simulink model "BLDCmotor_FOC_R2017b_fixdt"  (R2025a)
settings: Solver=FixedStepDiscrete  StartTime=0  StopTime=0.5  FixedStep=Ts  MaxStep=1e-6  RelTol=1e-6  AbsTol=1e-6  EnableMultiTasking=on
PreLoadFcn:
  | addpath(pwd);
  | addpath(genpath('01_Libraries'));
  | addpath(genpath('02_Figures'));
  | addpath(genpath('03_CreateParamTable'));
InitFcn:
  | init_model;
values from neighbouring files (symbols this model uses):
  a_cpr = 65535    [init_model.m]
  a_elecAngle = 60    [init_model.m]
  a_elecoffset = a_elecPeriod/12    (= 30)    [init_model.m]
  a_elecPeriod = 360    [init_model.m]
  a_fcpr = 1/65535    (= 1.52590218967e-05)    [init_model.m]
  a_mechoffset = a_elecoffset/n_polePairs    (= 5)    [init_model.m]
  a_phaAdvMax = 25    [init_model.m]
  b_angleMeasEna = 1    [init_model.m]
  b_cruiseCtrlEna = 0    [init_model.m]
  b_diagEna = 0    [init_model.m]
  b_fieldWeakEna = 0    [init_model.m]
  cf_currFilt = 0.692    [init_model.m]
  cf_idKi = Ki / (f_ctrl)    (= 0.00409061543436)    [init_model.m]
  cf_idKp = Kp    (= 0.0523598775598)    [init_model.m]
  cf_iqKi = Ki / (f_ctrl)    (= 0.00409061543436)    [init_model.m]
  cf_iqKiLimProt = 60 / (f_ctrl)    (= 0.00375)    [init_model.m]
  cf_iqKp = Kp    (= 0.0523598775598)    [init_model.m]
  cf_KbLimProt = Simulink.Parameter    [init_model.m]
  cf_nKi = 20.4 / (f_ctrl)    (= 0.001275)    [init_model.m]
  cf_nKiLimProt = 20 / (f_ctrl)    (= 0.00125)    [init_model.m]
  cf_nKp = 1.18    [init_model.m]
  cf_speedCoef = round(f_ctrl * a_mechAngle * (pi/180) * (30/pi))    [init_model.m]
  CTRL_FOC = 2    [init_model.m]
  CTRL_SIN = 1    [init_model.m]
  dV_openRate = 1000 / (f_ctrl)    (= 0.0625)    [init_model.m]
  dz_cntTrnsDetHi = 40    [init_model.m]
  dz_cntTrnsDetLo = 20    [init_model.m]
  ff_gain = ((r_motn / i_sca) * ((GD32_Vd_max_margin) / v_bus))    (= 0.338958333333)    [init_model.m]
  GD32_Vd_max_margin = GD32_Vd_max - V_margin    (= 1627)    [init_model.m]
  GD32_Vq_max_M1 = sqrt(GD32_Vd_max_margin^2 - GD32_Vq_max_XA.^2)    [init_model.m]
  i_max = i_max * i_sca    (= 500)    [init_model.m]
  id_fieldWeakMax = 5 * i_sca    (= 250)    [init_model.m]
  iq_maxSca_M1 = sqrt(1 - iq_maxSca_XA.^2)    [init_model.m]
  mcu_model = GD32F103    (= 1)    [init_model.m]
  n_commAcvLo = 15    [init_model.m]
  n_commDeacvHi = 30    [init_model.m]
  n_cruiseMotTgt = 0    [init_model.m]
  n_fieldWeakAuthHi = 300    [init_model.m]
  n_fieldWeakAuthLo = 100    [init_model.m]
  n_max = 1950    [init_model.m]
  n_polePairs = 6    [init_model.m]
  n_stdStillDet = 3    [init_model.m]
  OPEN_MODE = 0    [init_model.m]
  r_cos_M1 = cos((a_elecAngle_XA + a_elecPeriod/12)*(pi/180))    [init_model.m]
  r_errInpTgtThres = 600    [init_model.m]
  r_fieldWeakHi = 1000    [init_model.m]
  r_fieldWeakLo = 750    [init_model.m]
  r_motn = r_mot/2    (= 0.25)    [init_model.m]
  r_sin3PhaA_M1 = sin3Arm + A*r_sinPhaA_M1    [init_model.m]
  r_sin3PhaB_M1 = sin3Arm + A*r_sinPhaB_M1    [init_model.m]
  r_sin3PhaC_M1 = sin3Arm + A*r_sinPhaC_M1    [init_model.m]
  r_sin_M1 = sin((a_elecAngle_XA + a_elecPeriod/12)*(pi/180))    [init_model.m]
  SPD_MODE = 2    [init_model.m]
  STM32_Vd_max_margin = STM32_Vd_max - V_margin    (= 940)    [init_model.m]
  STM32_Vq_max_M1 = sqrt(STM32_Vd_max_margin^2 - STM32_Vq_max_XA.^2)    [init_model.m]
  t_errDequal = 1.80 * f_ctrl    (= 28800)    [init_model.m]
  t_errQual = 0.24 * f_ctrl    (= 3840)    [init_model.m]
  tgt_scale = 2047    [init_model.m]
  TRQ_MODE = 3    [init_model.m]
  Ts = 5e-6    (= 5e-06)    [init_model.m]
  Ts_ctrl = 6e-5    (= 6e-05)    [init_model.m]
  v_bus = 24    [init_model.m]
  vec_hallToPos = [0 2 0 1 4 3 5 0]    [init_model.m]
  VLT_MODE = 1    [init_model.m]
  z_commutMap_M1 = [-1 -1  0  1  1  0 ... (first row only)    [init_model.m]
  z_ctrlModReq = TRQ_MODE    (= 3)    [init_model.m]
  z_ctrlTypSel = CTRL_FOC    (= 2)    [init_model.m]
  z_maxCntRst = 2000    [init_model.m]
  z_selPhaCurMeasABC = 2    [init_model.m]
undefined symbols (not defined in the file or in its folder): BLDCmotor_FOC_R2017b_fixdt, DiscIntNeverNeededParam, DWORK0, DWORK1, DWORK2, DWORK3, powergui, spspowerguiLib
libraries: BLDC_controller_Lib x18, simulink x13, prociolib x6, eePwmGenerator x6, eePwmGeneratorMultilevel x3, mcbpositiondecoderlib x2, slpidlib x2, spsControlledVoltageSourceLib x1, spsMultimeterLib x1, spsPermanentMagnetSynchronousMachineLib x1, spsUniversalBridgeLib x1, spsVoltageMeasurementLib x1
(part 3 of 6)

== system BLDCmotor_FOC_R2017b_fixdt/BLDC_model_closed/__OutputSSForSFun__ ==
  __UniqueInportName__1__ : Inport
  __UniqueInportName__2__ : Inport  Port=2
  __UniqueInportName__3__ : Inport  Port=3
  __UniqueInportName__4__ : Inport  Port=4
  __UniqueInportName__5__ : Inport  Port=5
  __UniqueInportName__6__ : Inport  Port=6
  __UniqueInportName__7__ : Inport  Port=7
  __UniqueInportName__8__ : Inport  Port=8
  __UniqueInportName__9__ : Inport  Port=9
  __UniqueInportName__10__ : Inport  Port=10
  __UniqueInportName__11__ : Inport  Port=11
  __UniqueInportName__12__ : Inport  Port=12
  Mux1 : BusCreator  Inputs=12
  motor_out : Outport  VectorParamsAs1DForOutWhenUnconnected=off
  wires:
  __UniqueInportName__1__/1 -> Mux1/1  "Stator current is_a (A)"
  __UniqueInportName__2__/1 -> Mux1/2  "Stator current is_b (A)"
  __UniqueInportName__3__/1 -> Mux1/3  "Stator current is_c (A)"
  __UniqueInportName__4__/1 -> Mux1/4  "Stator back EMF e_a (V)"
  __UniqueInportName__5__/1 -> Mux1/5  "Stator back EMF e_b (V)"
  __UniqueInportName__6__/1 -> Mux1/6  "Stator back EMF e_cV)"
  __UniqueInportName__7__/1 -> Mux1/7  "Hall effect signal h_a"
  __UniqueInportName__8__/1 -> Mux1/8  "Hall effect signal h_b"
  __UniqueInportName__9__/1 -> Mux1/9  "Hall effect signal h_c"
  __UniqueInportName__10__/1 -> Mux1/10  "Rotor speed wm (rad/s)"
  __UniqueInportName__11__/1 -> Mux1/11  "Rotor angle thetam (rad)"
  __UniqueInportName__12__/1 -> Mux1/12  "Electromagnetic torque Te (N*m)"
  Mux1/1 -> motor_out/1

== system BLDCmotor_FOC_R2017b_fixdt/BLDC_model_open1/powergui ==
  note: Graphical user interface for the analysis of
      | Simscape Power Systems (Specialized Technology) circuits.
      | Place the Powergui block in the top-level of your model and double-click
      | on it to open the GUI.
  EquivalentModel1 : Subsystem
      mask init:
      | S  = GetDataForEquivalentModel('Discrete',gcbh);
      mask Display:
      | color('red')
      | disp('EQUIVALENT CIRCUIT\nDiscrete')
  Ground : Ground
  Terminator : Terminator
  wires:
  Ground/1 -> Terminator/1

== system BLDCmotor_FOC_R2017b_fixdt/PWM_gates/MCU_VD_Selector ==
  In1 : Inport
  Default_Control_Type : Subsystem
  Default_Control_Type1 : Subsystem
  If1 : If  IfExpression=u1 == 1
  Merge : Merge
  Vd_max1 : Constant  Value=GD32_Vd_max_margin  OutDataTypeStr=fixdt(1,16,4)
  Vd_max3 : Constant  Value=STM32_Vd_max_margin  OutDataTypeStr=fixdt(1,16,4)
  Out1 : Outport
  wires:
  Default_Control_Type/1(2) -> Merge/2
  Vd_max1/1 -> Default_Control_Type1/1(1)
  If1/2 -> Default_Control_Type/Action
  If1/1 -> Default_Control_Type1/Action
  Vd_max3/1 -> Default_Control_Type/1(1)
  In1/1 -> If1/1
  Merge/1 -> Out1/1
  Default_Control_Type1/1(2) -> Merge/1

== system BLDCmotor_FOC_R2017b_fixdt/PWM_gates/PWM_generator1 ==
  DC : Inport  SampleTime=Ts
  PWM_generator_sfcn : S-Function  FunctionName=PWM_generator_sf  SFunctionModules=""  SFunctionDeploymentMode=off  EnableBusSupport=off  SFcnStateName=DWORK0  mask{rtw_sf_name=PWM_generator_sf, showVar=off}
      mask prompts: rtw_sf_name "Simulink:masks:GenSFuncName_MP"; showVar "Simulink:masks:GenSFuncShowModuleList_MP"
      mask help: Simulink:masks:GenSFuncDesc_MD
      mask init: same as BLDCmotor_FOC_R2017b_fixdt/BLDC_model_closed/BLDC_model_sfcn
      settings: SFcnIsStateOwnerBlock=on
      settings: CopyFcn=|
      | if ~strcmp(get_param(gcb,'Linkstatus'),'none') && ...
      | ~strcmp(get_param(gcb,'Linkstatus'),'implicit')
      |   set_param(gcb,'LinkStatus','none');
      | end
      mask Help: eval('feval(''rtwprivate'',''rtwhelpview'',''rtw_sfcn_block'')');
      mask Display:
      | port_label('input',1,'DC');
      | port_label('output',1,'PWM');
  __InputSSForSFun__ : Subsystem
  __OutputSSForSFun__ : Subsystem
  PWM : Outport  VectorParamsAs1DForOutWhenUnconnected=off
  wires:
  __OutputSSForSFun__/1(PWM) -> PWM/1
  PWM_generator_sfcn/1 -> __OutputSSForSFun__/1(__UniqueInportName__1__)
  __InputSSForSFun__/1(__UniqueOutportName__1__) -> PWM_generator_sfcn/1
  DC/1 -> __InputSSForSFun__/1(DC)

== system BLDCmotor_FOC_R2017b_fixdt/PWM_gates/PWM_generator12 ==
  DC : Inport  SampleTime=Ts
  PWM_generator_sfcn : S-Function  FunctionName=PWM_generator_sf  SFunctionModules=""  SFunctionDeploymentMode=off  EnableBusSupport=off  SFcnStateName=DWORK0  mask{rtw_sf_name=PWM_generator_sf, showVar=off}
      mask prompts: rtw_sf_name "Simulink:masks:GenSFuncName_MP"; showVar "Simulink:masks:GenSFuncShowModuleList_MP"
      mask help: Simulink:masks:GenSFuncDesc_MD
      mask init: same as BLDCmotor_FOC_R2017b_fixdt/BLDC_model_closed/BLDC_model_sfcn
      settings: SFcnIsStateOwnerBlock=on
      settings: CopyFcn=|
      | if ~strcmp(get_param(gcb,'Linkstatus'),'none') && ...
      | ~strcmp(get_param(gcb,'Linkstatus'),'implicit')
      |   set_param(gcb,'LinkStatus','none');
      | end
      mask Help: eval('feval(''rtwprivate'',''rtwhelpview'',''rtw_sfcn_block'')');
      mask Display:
      | port_label('input',1,'DC');
      | port_label('output',1,'PWM');
  __InputSSForSFun__ : Subsystem
  __OutputSSForSFun__ : Subsystem
  PWM : Outport  VectorParamsAs1DForOutWhenUnconnected=off
  wires:
  DC/1 -> __InputSSForSFun__/1(DC)
  __InputSSForSFun__/1(__UniqueOutportName__1__) -> PWM_generator_sfcn/1
  PWM_generator_sfcn/1 -> __OutputSSForSFun__/1(__UniqueInportName__1__)
  __OutputSSForSFun__/1(PWM) -> PWM/1

== system BLDCmotor_FOC_R2017b_fixdt/PWM_gates/PWM_generator2 ==
  DC : Inport  SampleTime=Ts
  PWM_generator_sfcn : S-Function  FunctionName=PWM_generator_sf  SFunctionModules=""  SFunctionDeploymentMode=off  EnableBusSupport=off  SFcnStateName=DWORK0  mask{rtw_sf_name=PWM_generator_sf, showVar=off}
      mask prompts: rtw_sf_name "Simulink:masks:GenSFuncName_MP"; showVar "Simulink:masks:GenSFuncShowModuleList_MP"
      mask help: Simulink:masks:GenSFuncDesc_MD
      mask init: same as BLDCmotor_FOC_R2017b_fixdt/BLDC_model_closed/BLDC_model_sfcn
      settings: SFcnIsStateOwnerBlock=on
      settings: CopyFcn=|
      | if ~strcmp(get_param(gcb,'Linkstatus'),'none') && ...
      | ~strcmp(get_param(gcb,'Linkstatus'),'implicit')
      |   set_param(gcb,'LinkStatus','none');
      | end
      mask Help: eval('feval(''rtwprivate'',''rtwhelpview'',''rtw_sfcn_block'')');
      mask Display:
      | port_label('input',1,'DC');
      | port_label('output',1,'PWM');
  __InputSSForSFun__ : Subsystem
  __OutputSSForSFun__ : Subsystem
  PWM : Outport  VectorParamsAs1DForOutWhenUnconnected=off
  wires:
  DC/1 -> __InputSSForSFun__/1(DC)
  __InputSSForSFun__/1(__UniqueOutportName__1__) -> PWM_generator_sfcn/1
  PWM_generator_sfcn/1 -> __OutputSSForSFun__/1(__UniqueInportName__1__)
  __OutputSSForSFun__/1(PWM) -> PWM/1

== system BLDCmotor_FOC_R2017b_fixdt/PWM_gates/PWM_generator3 ==
  DC : Inport  SampleTime=Ts
  PWM_generator_sfcn : S-Function  FunctionName=PWM_generator_sf  SFunctionModules=""  SFunctionDeploymentMode=off  EnableBusSupport=off  SFcnStateName=DWORK0  mask{rtw_sf_name=PWM_generator_sf, showVar=off}
      mask prompts: rtw_sf_name "Simulink:masks:GenSFuncName_MP"; showVar "Simulink:masks:GenSFuncShowModuleList_MP"
      mask help: Simulink:masks:GenSFuncDesc_MD
      mask init: same as BLDCmotor_FOC_R2017b_fixdt/BLDC_model_closed/BLDC_model_sfcn
      settings: SFcnIsStateOwnerBlock=on
      settings: CopyFcn=|
      | if ~strcmp(get_param(gcb,'Linkstatus'),'none') && ...
      | ~strcmp(get_param(gcb,'Linkstatus'),'implicit')
      |   set_param(gcb,'LinkStatus','none');
      | end
      mask Help: eval('feval(''rtwprivate'',''rtwhelpview'',''rtw_sfcn_block'')');
      mask Display:
      | port_label('input',1,'DC');
      | port_label('output',1,'PWM');
  __InputSSForSFun__ : Subsystem
  __OutputSSForSFun__ : Subsystem
  PWM : Outport  VectorParamsAs1DForOutWhenUnconnected=off
  wires:
  __OutputSSForSFun__/1(PWM) -> PWM/1
  PWM_generator_sfcn/1 -> __OutputSSForSFun__/1(__UniqueInportName__1__)
  __InputSSForSFun__/1(__UniqueOutportName__1__) -> PWM_generator_sfcn/1
  DC/1 -> __InputSSForSFun__/1(DC)

== system BLDCmotor_FOC_R2017b_fixdt/PWM_gates/PWM_generator4 ==
  DC : Inport  SampleTime=Ts
  PWM_generator_sfcn : S-Function  FunctionName=PWM_generator_sf  SFunctionModules=""  SFunctionDeploymentMode=off  EnableBusSupport=off  SFcnStateName=DWORK0  mask{rtw_sf_name=PWM_generator_sf, showVar=off}
      mask prompts: rtw_sf_name "Simulink:masks:GenSFuncName_MP"; showVar "Simulink:masks:GenSFuncShowModuleList_MP"
      mask help: Simulink:masks:GenSFuncDesc_MD
      mask init: same as BLDCmotor_FOC_R2017b_fixdt/BLDC_model_closed/BLDC_model_sfcn
      settings: SFcnIsStateOwnerBlock=on
      settings: CopyFcn=|
      | if ~strcmp(get_param(gcb,'Linkstatus'),'none') && ...
      | ~strcmp(get_param(gcb,'Linkstatus'),'implicit')
      |   set_param(gcb,'LinkStatus','none');
      | end
      mask Help: eval('feval(''rtwprivate'',''rtwhelpview'',''rtw_sfcn_block'')');
      mask Display:
      | port_label('input',1,'DC');
      | port_label('output',1,'PWM');
  __InputSSForSFun__ : Subsystem
  __OutputSSForSFun__ : Subsystem
  PWM : Outport  VectorParamsAs1DForOutWhenUnconnected=off
  wires:
  DC/1 -> __InputSSForSFun__/1(DC)
  __InputSSForSFun__/1(__UniqueOutportName__1__) -> PWM_generator_sfcn/1
  PWM_generator_sfcn/1 -> __OutputSSForSFun__/1(__UniqueInportName__1__)
  __OutputSSForSFun__/1(PWM) -> PWM/1

== system BLDCmotor_FOC_R2017b_fixdt/PWM_gates/PWM_generator5 ==
  DC : Inport  SampleTime=Ts
  PWM_generator_sfcn : S-Function  FunctionName=PWM_generator_sf  SFunctionModules=""  SFunctionDeploymentMode=off  EnableBusSupport=off  SFcnStateName=DWORK0  mask{rtw_sf_name=PWM_generator_sf, showVar=off}
      mask prompts: rtw_sf_name "Simulink:masks:GenSFuncName_MP"; showVar "Simulink:masks:GenSFuncShowModuleList_MP"
      mask help: Simulink:masks:GenSFuncDesc_MD
      mask init: same as BLDCmotor_FOC_R2017b_fixdt/BLDC_model_closed/BLDC_model_sfcn
      settings: SFcnIsStateOwnerBlock=on
      settings: CopyFcn=|
      | if ~strcmp(get_param(gcb,'Linkstatus'),'none') && ...
      | ~strcmp(get_param(gcb,'Linkstatus'),'implicit')
      |   set_param(gcb,'LinkStatus','none');
      | end
      mask Help: eval('feval(''rtwprivate'',''rtwhelpview'',''rtw_sfcn_block'')');
      mask Display:
      | port_label('input',1,'DC');
      | port_label('output',1,'PWM');
  __InputSSForSFun__ : Subsystem
  __OutputSSForSFun__ : Subsystem
  PWM : Outport  VectorParamsAs1DForOutWhenUnconnected=off
  wires:
  __OutputSSForSFun__/1(PWM) -> PWM/1
  PWM_generator_sfcn/1 -> __OutputSSForSFun__/1(__UniqueInportName__1__)
  __InputSSForSFun__/1(__UniqueOutportName__1__) -> PWM_generator_sfcn/1
  DC/1 -> __InputSSForSFun__/1(DC)

== system BLDCmotor_FOC_R2017b_fixdt/PWM_gates/signal_log6 ==
  PWM : Inport
  Terminator_1 : Terminator
  wires:
  PWM/1 -> Terminator_1/1  "PWM"

== system BLDCmotor_FOC_R2017b_fixdt/Power Stage/Subsystem ==
  the : Inport
  Angle converter : spsPMSynchronousMachineModel/Discrete/Hall effect sensor/Angle converter  SystemSampleTime=-1  VariantActivationTime=update diagram  EmptyChoice=off  PassThrough=off  PassThroughVariantControl=(default)  EmptyChoiceVariantControl=(default)  AllowFlexibleInterface=on  Latency=0  AutoFrameSizeCalculation=off
  Bus Creator : BusCreator  Inputs=3
  Constant : Constant  Value=-60
  Constant1 : Constant  Value=120
  Constant2 : Constant  Value=60
  Constant3 : Constant  Value=-120
  Constant4 : Constant  Value=-180
  Constant5 : Constant  Value=0
  Data Type Conversion : DataTypeConversion  OutDataTypeStr=double
  Data Type Conversion1 : DataTypeConversion  OutDataTypeStr=double
  Data Type Conversion2 : DataTypeConversion  OutDataTypeStr=double
  Logical Operator : Logic  AllPortsSameDT=off  OutDataTypeStr=boolean
  Logical Operator1 : Logic  Operator=OR  AllPortsSameDT=off  OutDataTypeStr=boolean
  Logical Operator2 : Logic  AllPortsSameDT=off  OutDataTypeStr=boolean
  Relational Operator1 : RelationalOperator  Operator=<=
  Relational Operator2 : RelationalOperator
  Relational Operator3 : RelationalOperator  Operator=<=
  Relational Operator4 : RelationalOperator
  Relational Operator5 : RelationalOperator  Operator=<=
  Relational Operator6 : RelationalOperator
  Hall : Outport  VectorParamsAs1DForOutWhenUnconnected=off
  wires:
  Relational Operator4/1 -> Logical Operator1/1
  Constant/1 -> Relational Operator2/2
  Logical Operator/1 -> Data Type Conversion/1
  Logical Operator1/1 -> Data Type Conversion1/1
  Relational Operator5/1 -> Logical Operator2/2
  Angle converter/1 -> Relational Operator2/1, Relational Operator1/1, Relational Operator6/1, Relational Operator5/1, Relational Operator3/1, Relational Operator4/1
  Logical Operator2/1 -> Data Type Conversion2/1
  Constant2/1 -> Relational Operator4/2
  Data Type Conversion1/1 -> Bus Creator/2
  the/1 -> Angle converter/1
  Data Type Conversion/1 -> Bus Creator/1
  Constant5/1 -> Relational Operator5/2
  Data Type Conversion2/1 -> Bus Creator/3
  Relational Operator3/1 -> Logical Operator1/2
  Constant4/1 -> Relational Operator6/2
  Relational Operator1/1 -> Logical Operator/2
  Relational Operator2/1 -> Logical Operator/1
  Relational Operator6/1 -> Logical Operator2/1
  Bus Creator/1 -> Hall/1
  Constant3/1 -> Relational Operator3/2
  Constant1/1 -> Relational Operator1/2

== system BLDCmotor_FOC_R2017b_fixdt/Power Stage/Variant Subsystem ==
  note: 1) Add Subsystem or Model blocks as valid variant choices.
      | 2) You cannot connect blocks at this level. At simulation, connectivity is automatically
      | determined, based on the active variant and port name matching.
  GD32F103 : Subsystem  TreatAsAtomicUnit=on  VariantControl=mcu_model == 1
  STM32F103 : Subsystem  TreatAsAtomicUnit=on  VariantControl=mcu_model == 0
  Vd_max_margin : Outport

== system BLDCmotor_FOC_R2017b_fixdt/filtLowPass/Low_Pass_Filter ==
  u : Inport
  coef : Inport  Port=2
  Divide3 : Product  Inputs=**  OutDataTypeStr=fixdt(1,32,16)  RndMeth=Simplest  SaturateOnIntegerOverflow=on
  Scope1 : Scope  NumInputPorts=3
      settings: ActiveDisplayYMinimum=-7973.4546189633093  ActiveDisplayYMaximum=13277.671743224013
  Sum2 : Sum  Inputs=+-  RndMeth=Simplest
  Sum3 : Sum  RndMeth=Simplest  OutDataTypeStr=Inherit: Same as first input
  UnitDelay1 : UnitDelay  SampleTime=-1  HasFrameUpgradeWarning=on
  y : Outport  VectorParamsAs1DForOutWhenUnconnected=off
  wires:
  Divide3/1 -> Scope1/2, Sum3/1
  Sum3/1 -> y/1, Scope1/3, UnitDelay1/1
  UnitDelay1/1 -> Sum3/2, Sum2/2
  Sum2/1 -> Divide3/1, Scope1/1
  u/1 -> Sum2/1
  coef/1 -> Divide3/2

== system BLDCmotor_FOC_R2017b_fixdt/rateLimiter/Rate_Limiter ==
  note: Rate Limiter
      | Note: The sample time must be included in the Increment and Decrement values.
  u : Inport
  inc : Inport  Port=2
  dec : Inport  Port=3
  Saturation Dynamic : simulink/Discontinuities/Saturation Dynamic  OutMin=[]  OutMax=[]  OutDataTypeStr=Inherit: Same as second input  OutDataType=fixdt(1, 16)  OutScaling=2^-10  DoSatur=off
  Sum1 : Sum  Inputs=+-  RndMeth=Zero  OutDataTypeStr=Inherit: Same as first input
  Sum2 : Sum  RndMeth=Zero  OutDataTypeStr=Inherit: Same as first input
  UnitDelay : UnitDelay  SampleTime=-1  HasFrameUpgradeWarning=on
      settings: AttributesFormatString=Ini=%<X0>
  y : Outport  VectorParamsAs1DForOutWhenUnconnected=off
  wires:
  Saturation Dynamic/1 -> Sum2/1
  dec/1 -> Saturation Dynamic/3
  Sum1/1 -> Saturation Dynamic/2
  Sum2/1 -> UnitDelay/1, y/1
  inc/1 -> Saturation Dynamic/1
  u/1 -> Sum1/1
  UnitDelay/1 -> Sum2/2, Sum1/2

== system BLDCmotor_FOC_R2017b_fixdt/BLDC_controller/F01_Estimations/F01_01_Edge_Detector ==
  b_hallA : Inport
  b_hallB : Inport  Port=2
  b_hallC : Inport  Port=3
  Logical Operator : Logic  Operator=XOR  Inputs=6  AllPortsSameDT=off  OutDataTypeStr=boolean
  UnitDelay1 : UnitDelay  SampleTime=-1  HasFrameUpgradeWarning=on
      settings: AttributesFormatString=Ini=%<X0>
  UnitDelay2 : UnitDelay  SampleTime=-1  HasFrameUpgradeWarning=on
      settings: AttributesFormatString=Ini=%<X0>
  UnitDelay3 : UnitDelay  SampleTime=-1  HasFrameUpgradeWarning=on
      settings: AttributesFormatString=Ini=%<X0>
  "b_edge " : Outport  OutputWhenDisabled=reset  InitialOutput=0  VectorParamsAs1DForOutWhenUnconnected=off
  wires:
  b_hallA/1 -> Logical Operator/1, UnitDelay3/1
  b_hallC/1 -> Logical Operator/3, UnitDelay2/1
  b_hallB/1 -> Logical Operator/2, UnitDelay1/1
  UnitDelay1/1 -> Logical Operator/5
  UnitDelay2/1 -> Logical Operator/6
  UnitDelay3/1 -> Logical Operator/4
  Logical Operator/1 -> "b_edge "/1

== system BLDCmotor_FOC_R2017b_fixdt/BLDC_controller/F01_Estimations/F01_02_Position_Calculation ==
  note: This calculates the low resolution position based on Hall sensors.
  b_hallA : Inport
  b_hallB : Inport  Port=2
  b_hallC : Inport  Port=3
  Selector : Selector  IndexMode=Zero-based  InputPortWidth=length(vec_hallToPos)  IndexOptions=Index vector (port)  Indices=[1 3]  OutputSizes=1
  Sum : Sum  Inputs=+++  RndMeth=Simplest  OutDataTypeStr=Inherit: Same as first input
  g_Ha : Gain  Gain=4  OutDataTypeStr=Inherit: Inherit via back propagation  RndMeth=Zero  ParamDataTypeStr=Inherit: Same as input
  g_Hb : Gain  Gain=2  OutDataTypeStr=Inherit: Inherit via back propagation  RndMeth=Simplest  ParamDataTypeStr=Inherit: Same as input
  vec_hallToPos : Constant  Value=vec_hallToPos  OutDataTypeStr=int8
  z_posRaw : Outport  OutputWhenDisabled=reset  InitialOutput=0  VectorParamsAs1DForOutWhenUnconnected=off
  "z_pos " : Outport  Port=2  OutputWhenDisabled=reset  InitialOutput=0  VectorParamsAs1DForOutWhenUnconnected=off
  wires:
  b_hallC/1 -> Sum/3
  g_Ha/1 -> Sum/1
  g_Hb/1 -> Sum/2
  Sum/1 -> z_posRaw/1, Selector/2
  b_hallA/1 -> g_Ha/1
  b_hallB/1 -> g_Hb/1
  vec_hallToPos/1 -> Selector/1
  Selector/1 -> "z_pos "/1

== system BLDCmotor_FOC_R2017b_fixdt/BLDC_controller/F01_Estimations/F01_03_Direction_Detection ==
  z_pos : Inport
  Action Port : ActionPort  ActionPortLabel=if(u1 ~= 0)
  Constant20 : Constant  Value=-5  OutDataTypeStr=Inherit: Inherit via back propagation
  Constant23 : Constant  Value=-1  OutDataTypeStr=int8
  Constant24 : Constant  OutDataTypeStr=int8
  Constant8 : Constant  OutDataTypeStr=Inherit: Inherit via back propagation
  Logical Operator3 : Logic  Operator=OR  AllPortsSameDT=off  OutDataTypeStr=boolean
  Relational Operator1 : RelationalOperator  Operator===  OutDataTypeStr=boolean  RndMeth=Simplest  InputSameDT=off
  Relational Operator6 : RelationalOperator  Operator===  OutDataTypeStr=boolean  RndMeth=Simplest  InputSameDT=off
  Sum2 : Sum  Inputs=|+-  InputSameDT=on  RndMeth=Zero  OutDataTypeStr=Inherit: Same as first input
  Switch2 : Switch  Criteria=u2 ~= 0  OutDataTypeStr=Inherit: Inherit via back propagation  RndMeth=Simplest  SaturateOnIntegerOverflow=off  InputSameDT=off
  UnitDelay2 : UnitDelay  SampleTime=-1  HasFrameUpgradeWarning=on
  UnitDelay3 : UnitDelay  SampleTime=-1  HasFrameUpgradeWarning=on
      settings: AttributesFormatString=Ini=%<X0>
  z_dir : Outport  VectorParamsAs1DForOutWhenUnconnected=off
  z_dirPrev : Outport  Port=2  VectorParamsAs1DForOutWhenUnconnected=off
  wires:
  UnitDelay2/1 -> Sum2/2
  Relational Operator1/1 -> Logical Operator3/1
  Constant8/1 -> Relational Operator1/2
  Sum2/1 -> Relational Operator6/1, Relational Operator1/1
  Relational Operator6/1 -> Logical Operator3/2
  Constant20/1 -> Relational Operator6/2
  Constant24/1 -> Switch2/1
  Constant23/1 -> Switch2/3
  Logical Operator3/1 -> Switch2/2
  z_pos/1 -> Sum2/1, UnitDelay2/1
  Switch2/1 -> UnitDelay3/1, z_dir/1
  UnitDelay3/1 -> z_dirPrev/1

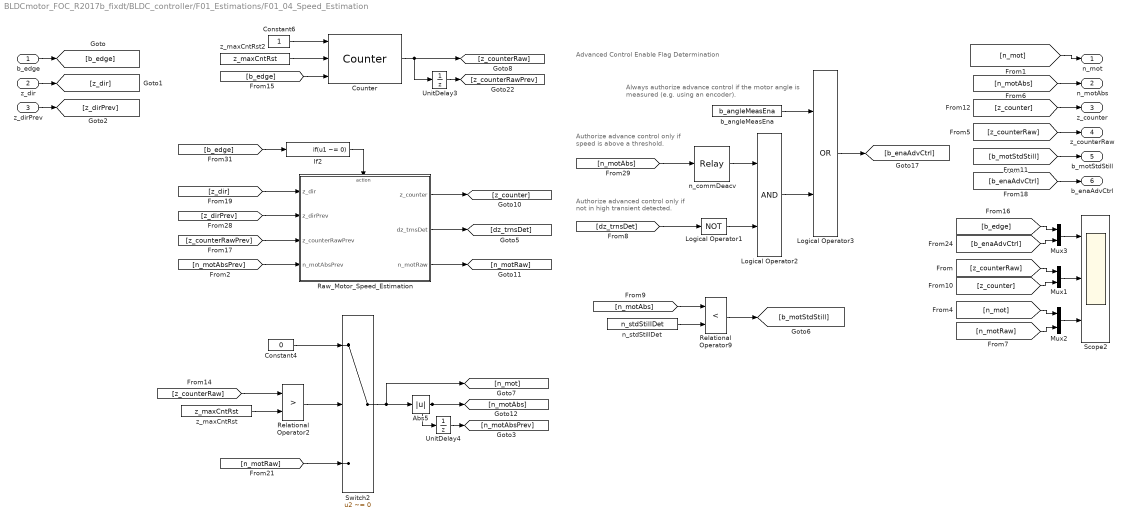
== system BLDCmotor_FOC_R2017b_fixdt/BLDC_controller/F01_Estimations/F01_04_Speed_Estimation ==
  note: Advanced Control Enable Flag Determination
  note: Authorize advance control only if speed is above a threshold.
  note: Authorize advanced control only if not in high transient detected.
  note: Always authorize advance control if the motor angle is measured (e.g. using an encoder).
  b_edge : Inport
  z_dir : Inport  Port=2
  z_dirPrev : Inport  Port=3
  Abs5 : Abs  OutDataTypeStr=Inherit: Inherit via back propagation  RndMeth=Zero  SaturateOnIntegerOverflow=off
  Constant4 : Constant  Value=0  OutDataTypeStr=Inherit: Inherit via back propagation
  Constant6 : Constant  OutDataTypeStr=fixdt(1,16,0)
  Counter : BLDC_controller_Lib/Counter  z_cntInit=z_maxCntRst
      settings: AttributesFormatString=Ini=%<z_cntInit>
  If2 : If  IfExpression=u1 ~= 0  ShowElse=off
  Logical Operator1 : Logic  Operator=NOT  AllPortsSameDT=off  OutDataTypeStr=boolean
  Logical Operator2 : Logic  AllPortsSameDT=off  OutDataTypeStr=boolean
  Logical Operator3 : Logic  Operator=OR  AllPortsSameDT=off  OutDataTypeStr=boolean
  Mux1 : Mux  Inputs=2
  Mux2 : Mux  Inputs=2
  Mux3 : Mux  Inputs=2
  Raw_Motor_Speed_Estimation : Subsystem
  Relational Operator2 : RelationalOperator  Operator=>  OutDataTypeStr=boolean  RndMeth=Simplest  InputSameDT=off
  Relational Operator9 : RelationalOperator  Operator=<  OutDataTypeStr=boolean  RndMeth=Simplest  InputSameDT=off
  Scope2 : Scope  NumInputPorts=3
      settings: ActiveDisplayYMinimum=-0.12499999999999997  ActiveDisplayYMaximum=1.125
  Switch2 : Switch  Criteria=u2 ~= 0  OutDataTypeStr=Inherit: Inherit via back propagation  RndMeth=Zero  SaturateOnIntegerOverflow=off  InputSameDT=off
  UnitDelay3 : UnitDelay  InitialCondition=z_maxCntRst  SampleTime=-1  HasFrameUpgradeWarning=on
      settings: AttributesFormatString=Ini=%<X0>
  UnitDelay4 : UnitDelay  SampleTime=-1  HasFrameUpgradeWarning=on
      settings: AttributesFormatString=Ini=%<X0>
  b_angleMeasEna : Constant  Value=b_angleMeasEna  OutDataTypeStr=boolean
  n_commDeacv : Relay  OnSwitchValue=n_commDeacvHi  OffSwitchValue=n_commAcvLo  OutDataTypeStr=boolean
  n_stdStillDet : Constant  Value=n_stdStillDet  OutDataTypeStr=Inherit: Inherit via back propagation
  z_maxCntRst : Constant  Value=z_maxCntRst  OutDataTypeStr=Inherit: Inherit via back propagation
  z_maxCntRst2 : Constant  Value=z_maxCntRst  OutDataTypeStr=Inherit: Inherit via back propagation
  n_mot : Outport  VectorParamsAs1DForOutWhenUnconnected=off
  n_motAbs : Outport  Port=2  VectorParamsAs1DForOutWhenUnconnected=off
  z_counter : Outport  Port=3  OutputWhenDisabled=reset  InitialOutput=0  VectorParamsAs1DForOutWhenUnconnected=off
  z_counterRaw : Outport  Port=4  OutputWhenDisabled=reset  InitialOutput=0  VectorParamsAs1DForOutWhenUnconnected=off
  b_motStdStill : Outport  Port=5  OutputWhenDisabled=reset  InitialOutput=0  VectorParamsAs1DForOutWhenUnconnected=off
  b_enaAdvCtrl : Outport  Port=6  VectorParamsAs1DForOutWhenUnconnected=off
  wires:
  [n_motRaw] -> Mux2/2
  Mux2/1 -> Scope2/3
  [n_mot] -> Mux2/1
  Mux1/1 -> Scope2/2
  [z_counterRaw] -> Mux1/1
  [z_counter] -> Mux1/2
  b_edge/1 -> [b_edge]
  [n_mot] -> n_mot/1
  z_dir/1 -> [z_dir]
  [z_counter] -> z_counter/1
  [z_counterRaw] -> z_counterRaw/1
  UnitDelay3/1 -> [z_counterRawPrev]
  z_dirPrev/1 -> [z_dirPrev]
  [z_dir] -> Raw_Motor_Speed_Estimation/1(z_dir)
  Abs5/1 -> UnitDelay4/1, [n_motAbs]
  Raw_Motor_Speed_Estimation/1(z_counter) -> [z_counter]
  [z_dirPrev] -> Raw_Motor_Speed_Estimation/2(z_dirPrev)
  If2/1 -> Raw_Motor_Speed_Estimation/Action
  [z_counterRawPrev] -> Raw_Motor_Speed_Estimation/3(z_counterRawPrev)
  [b_enaAdvCtrl] -> b_enaAdvCtrl/1
  [z_counterRaw] -> Relational Operator2/1
  z_maxCntRst/1 -> Relational Operator2/2
  Constant4/1 -> Switch2/1
  Raw_Motor_Speed_Estimation/3(n_motRaw) -> [n_motRaw]
  Switch2/1 -> [n_mot], Abs5/1
  Mux3/1 -> Scope2/1
  [b_enaAdvCtrl] -> Mux3/2
  [b_edge] -> Mux3/1
  [b_edge] -> If2/1
  Relational Operator2/1 -> Switch2/2
  UnitDelay4/1 -> [n_motAbsPrev]
  [n_motAbsPrev] -> Raw_Motor_Speed_Estimation/4(n_motAbsPrev)
  [n_motAbs] -> n_motAbs/1
  [n_motAbs] -> n_commDeacv/1
  Raw_Motor_Speed_Estimation/2(dz_trnsDet) -> [dz_trnsDet]
  n_commDeacv/1 -> Logical Operator2/1
  Logical Operator1/1 -> Logical Operator2/2
  [dz_trnsDet] -> Logical Operator1/1
  z_maxCntRst2/1 -> Counter/2
  [b_edge] -> Counter/3
  Constant6/1 -> Counter/1
  Counter/1 -> UnitDelay3/1, [z_counterRaw]
  [b_motStdStill] -> b_motStdStill/1
  [n_motAbs] -> Relational Operator9/1
  n_stdStillDet/1 -> Relational Operator9/2
  Relational Operator9/1 -> [b_motStdStill]
  [n_motRaw] -> Switch2/3
  Logical Operator3/1 -> [b_enaAdvCtrl]
  Logical Operator2/1 -> Logical Operator3/2
  b_angleMeasEna/1 -> Logical Operator3/1

== system BLDCmotor_FOC_R2017b_fixdt/BLDC_controller/F01_Estimations/F01_05_Electrical_Angle_Estimation ==
  note: Electrical angle calculation
  note: This switch is to manage the situation when FOC control method is not enabled.
  note: Electrical angle calculation:
      | a_elecAngle = a_elecAngle_C * (z_posLowRes + z_dir * (z_counterRaw / z_counter))
      | where a_elecAngle_C = 60
      | The min, max are for protection against angle overflow.
  z_pos : Inport
  z_dir : Inport  Port=2
  z_counter : Inport  Port=3
  z_counterRaw : Inport  Port=4
  b_enaAdvCtrl : Inport  Port=5
  Action Port : ActionPort  ActionPortLabel=if(u1 == 0)
  Constant1 : Constant  Value=0  OutDataTypeStr=Inherit: Inherit via back propagation
  Constant16 : Constant  OutDataTypeStr=Inherit: Inherit via back propagation
  Constant2 : Constant  OutDataTypeStr=Inherit: Inherit via back propagation
  Divide1 : Product  Inputs=*/  OutDataTypeStr=fixdt(1,16,14)  RndMeth=Simplest
  Divide2 : Product  Inputs=**  RndMeth=Simplest  OutDataTypeStr=Inherit: Same as first input
  Divide3 : Product  Inputs=**  RndMeth=Simplest  OutDataTypeStr=Inherit: Same as first input
  MinMax : MinMax  Inputs=2
  MinMax1 : MinMax  Function=max  Inputs=2
  Relational Operator7 : RelationalOperator  Operator===  OutDataTypeStr=boolean  RndMeth=Simplest  InputSameDT=off
  Scope : Scope  NumInputPorts=3
      settings: ActiveDisplayYMinimum=-45  ActiveDisplayYMaximum=405
  Signal Conversion2 : SignalConversion  OverrideOpt=off
  Sum1 : Sum  RndMeth=Simplest  OutDataTypeStr=Inherit: Same as first input
  Sum3 : Sum  OutDataTypeStr=fixdt(1,16,12)  RndMeth=Simplest
  Switch2 : Switch  Criteria=u2 ~= 0  OutDataTypeStr=Inherit: Inherit via back propagation  RndMeth=Zero  SaturateOnIntegerOverflow=off  InputSameDT=off
  Switch3 : Switch  Criteria=u2 ~= 0  OutDataTypeStr=Inherit: Inherit via back propagation  RndMeth=Zero  SaturateOnIntegerOverflow=off  InputSameDT=off
  a_elecAngle1 : Constant  Value=a_elecAngle  OutDataTypeStr=Inherit: Inherit via back propagation
  a_elecAngle : Outport  VectorParamsAs1DForOutWhenUnconnected=off
  wires:
  z_pos/1 -> [z_pos]
  z_dir/1 -> [z_dir]
  [a_elecAngle] -> Scope/1
  [b_enaAdvCtrl] -> Scope/3
  z_counterRaw/1 -> [z_counterRaw]
  z_counter/1 -> [z_counter]
  [z_pos] -> Switch3/1, Sum1/1
  Constant2/1 -> Sum1/2
  Relational Operator7/1 -> Switch3/2
  Constant16/1 -> Relational Operator7/2
  [z_dir] -> Relational Operator7/1
  Sum1/1 -> Switch3/3
  b_enaAdvCtrl/1 -> [b_enaAdvCtrl]
  [a_elecAngle] -> Signal Conversion2/1
  a_elecAngle1/1 -> Divide2/1
  [b_enaAdvCtrl] -> Switch2/2
  Sum3/1 -> [z_posHighRes], Switch2/1
  Divide3/1 -> Sum3/1
  Divide2/1 -> [a_elecAngle]
  [z_posLowRes] -> Sum3/2, Switch2/3
  Switch3/1 -> [z_posLowRes]
  [z_posHighRes] -> Scope/2
  Divide1/1 -> Divide3/1
  [z_dir] -> Divide3/2
  MinMax/1 -> Divide1/1
  [z_counterRaw] -> MinMax/1
  [z_counter] -> MinMax/2, Divide1/2
  Switch2/1 -> MinMax1/1
  Constant1/1 -> MinMax1/2
  MinMax1/1 -> Divide2/2
  Signal Conversion2/1 -> a_elecAngle/1

== system BLDCmotor_FOC_R2017b_fixdt/BLDC_controller/F01_Estimations/F01_06_Electrical_Angle_Measurement ==
  note: Shift angle with -30 deg to match the sin, cos look-up tables.
  note: Electrical angle calculation
  a_encoderCNT : Inport
  a_mechangle : Inport  Port=2
  Action Port : ActionPort  ActionPortLabel=else
  Constant : Constant  Value=a_cpr  OutDataTypeStr=fixdt(0,16,0)
  Constant1 : Constant  Value=a_mechoffset  OutDataTypeStr=uint16
  Constant2 : Constant  Commented=on  Value=a_elecoffset  OutDataTypeStr=Inherit: Inherit via back propagation
  Constant3 : Constant  Value=a_fcpr  OutDataTypeStr=fixdt(0,32,32)
  Data Type Conversion1 : DataTypeConversion  Commented=on  OutDataTypeStr=fixdt(0,16,0)  SaturateOnIntegerOverflow=off  RndMeth=Floor
  Data Type Conversion20 : DataTypeConversion  Commented=on  OutDataTypeStr=fixdt(1,16,6)  SaturateOnIntegerOverflow=off  RndMeth=Floor
  Divide : Product  Commented=on  Inputs=**
  From1 : From  Commented=on  GotoTag=a_mechangle
  Goto2 : Goto  Commented=on  GotoTag=a_mechangle
  Goto3 : Goto  Commented=on  GotoTag=a_elecAngle
  MechElec : Scope  NumInputPorts=7
      settings: ActiveDisplayYMinimum=-225.99465496649157  ActiveDisplayYMaximum=1430.7297186223789  DataLoggingVariableName=ScopeData4
  Mechanical to Electrical Position : mcbpositiondecoderlib/Mechanical to Electrical Position  PolePairsInputType=Input port  NrPP=n_polePairs  selectedRange=Degrees  MechOfstInputType=Input port  mechOffsetIn=a_mechoffset  maxAngleIn=360  InputDataType=fixdt(0,16,7)  VariantSelect=floating-point
      settings: LibrarySourceBlock=mcblib/Sensor Decoders/Mechanical to Electrical Position
  Modulo_fixdt : BLDC_controller_Lib/Modulo_fixdt  Commented=on  SystemSampleTime=-1  VariantActivationTime=update diagram  EmptyChoice=off  PassThrough=off  PassThroughVariantControl=(default)  EmptyChoiceVariantControl=(default)  AllowFlexibleInterface=on  Latency=0  AutoFrameSizeCalculation=off
  Quadrature Decoder : mcbpositiondecoderlib/Quadrature Decoder  ParameterInputType=on  CountsPerRevInverseDataType=fixdt(0,32,32)  EncoderSlitsPerRevolution=a_cpr  EncoderCountsPerSlit=1  CounterSize=16 bits  ExternalIndexCount=off  PositionUnit=Degrees  PositionDataType=fixdt(0,16,7)
      settings: LibrarySourceBlock=mcblib/Sensor Decoders/Quadrature Decoder
  Sum1 : Sum  Commented=on  Inputs=+-  RndMeth=Simplest  OutDataTypeStr=Inherit: Same as first input
  a_elecPeriod : Constant  Commented=on  Value=a_elecPeriod  OutDataTypeStr=Inherit: Inherit via back propagation
  n_polePairs : Constant  Commented=on  Value=n_polePairs  OutDataTypeStr=uint8
  n_polePairs1 : Constant  Value=n_polePairs  OutDataTypeStr=uint16
  a_elecAngle : Outport  VectorParamsAs1DForOutWhenUnconnected=off
  wires:
  [a_elecAngle] -> a_elecAngle/1
  a_encoderCNT/1 -> [a_encoderCNT]
  n_polePairs/1 -> Divide/2
  a_elecPeriod/1 -> Modulo_fixdt/2
  Constant2/1 -> Sum1/2
  Divide/1 -> Sum1/1
  Sum1/1 -> MechElec/4, Modulo_fixdt/1
  Modulo_fixdt/1 -> MechElec/3, Data Type Conversion20/1
  Quadrature Decoder/1 -> Mechanical to Electrical Position/1, MechElec/5
  From1/1 -> Divide/1, MechElec/1
  [a_encoderCNT] -> MechElec/7, Quadrature Decoder/1
  n_polePairs1/1 -> Mechanical to Electrical Position/2
  Mechanical to Electrical Position/1 -> MechElec/6, [a_elecAngle]
  a_mechangle/1 -> Goto2/1
  Data Type Conversion20/1 -> Goto3/1, MechElec/2
  Constant1/1 -> Mechanical to Electrical Position/3
  Constant/1 -> Quadrature Decoder/2
  Constant3/1 -> Quadrature Decoder/3

== system BLDCmotor_FOC_R2017b_fixdt/BLDC_controller/F02_Diagnostics/Diagnostics_Enabled ==
  note: Error 001: Hall sensor not connected
  note: Error 002: Hall sensor short circuit
  note: Error Qualification
  note: Error Detection
  note: Error Reporting
  note: Error 004: Motor NOT able to spin.
      |
      | Possible causes:
      | - motor phase disconnected
      | - MOSFET defective
      | - Operational Amplifier defective
      | - motor blocked
  note: This switch makes sure that once this error is SET, it can only be erased by a board restart cycle.
  note: If the Voltage applied to the motor is above a threshold but the motor does NOT spin, then there is an error.
      | Note: The error is checked only if the motor is Enabled. If it is Disabled it will not spin anyway.
  b_motEna : Inport
  z_posRaw : Inport  Port=2
  b_motStdStill : Inport  Port=3
  VqFinPrev : Inport  Port=4
  Action Port : ActionPort  ActionPortLabel=if(u1 ~= 0)
  Abs4 : Abs  SaturateOnIntegerOverflow=off
  Bitwise Operator1 : simulink/Logic and Bit Operations/Bitwise Operator  logicop=AND  UseBitMask=on  BitMask=bin2dec('100')  BitMaskRealWorld=Stored Integer
  CTRL_COMM : Constant  Value=0  OutDataTypeStr=Inherit: Inherit via back propagation
  CTRL_COMM1 : Constant  Value=7  OutDataTypeStr=Inherit: Inherit via back propagation
  CTRL_COMM2 : Constant  Value=0  OutDataTypeStr=Inherit: Inherit via back propagation
  CTRL_COMM4 : Constant  OutDataTypeStr=Inherit: Inherit via back propagation
  Data Type Conversion : DataTypeConversion  OutDataTypeStr=uint8  SaturateOnIntegerOverflow=off  RndMeth=Floor
  Data Type Conversion1 : DataTypeConversion  OutDataTypeStr=uint8  SaturateOnIntegerOverflow=off  RndMeth=Floor
  Data Type Conversion3 : DataTypeConversion  OutDataTypeStr=uint8  SaturateOnIntegerOverflow=off  RndMeth=Floor
  Debounce_Filter : BLDC_controller_Lib/Debounce_Filter
  Logical Operator1 : Logic  Inputs=3  AllPortsSameDT=off  OutDataTypeStr=boolean
  Relational Operator1 : RelationalOperator  Operator===  OutDataTypeStr=boolean  RndMeth=Simplest  InputSameDT=off
  Relational Operator2 : RelationalOperator  Operator=~=  OutDataTypeStr=boolean  RndMeth=Simplest  InputSameDT=off
  Relational Operator3 : RelationalOperator  Operator===  OutDataTypeStr=boolean  RndMeth=Simplest  InputSameDT=off
  Relational Operator7 : RelationalOperator  Operator=>  OutDataTypeStr=boolean  RndMeth=Simplest  InputSameDT=off
  Sum : Sum  Inputs=+++  RndMeth=Simplest  OutDataTypeStr=Inherit: Same as first input
  Switch1 : Switch  Criteria=u2 ~= 0  OutDataTypeStr=Inherit: Inherit via back propagation  RndMeth=Zero  SaturateOnIntegerOverflow=off  InputSameDT=off
  Switch3 : Switch  Criteria=u2 ~= 0  OutDataTypeStr=Inherit: Inherit via back propagation  RndMeth=Zero  SaturateOnIntegerOverflow=off  InputSameDT=off
  UnitDelay : UnitDelay  SampleTime=-1  HasFrameUpgradeWarning=on
      settings: AttributesFormatString=Ini=%<X0>
  either_edge : BLDC_controller_Lib/either_edge
  g_Hb : Gain  Gain=2  RndMeth=Simplest  OutDataTypeStr=Inherit: Same as input
  g_Hb1 : Gain  Gain=4  RndMeth=Simplest  OutDataTypeStr=Inherit: Same as input
  r_errInpTgtThres : Constant  Value=r_errInpTgtThres  OutDataTypeStr=Inherit: Inherit via back propagation
  t_errDequal : Constant  Value=t_errDequal  OutDataTypeStr=Inherit: Inherit via back propagation
  t_errQual : Constant  Value=t_errQual  OutDataTypeStr=Inherit: Inherit via back propagation
  "z_errCode " : Outport  VectorParamsAs1DForOutWhenUnconnected=off
  b_errFlag : Outport  Port=2  VectorParamsAs1DForOutWhenUnconnected=off
  wires:
  [z_errCode] -> "z_errCode "/1
  z_posRaw/1 -> [z_posRaw]
  t_errDequal/1 -> Debounce_Filter/3
  t_errQual/1 -> Debounce_Filter/2
  CTRL_COMM/1 -> Relational Operator3/2
  CTRL_COMM1/1 -> Relational Operator1/2
  [z_posRaw] -> Relational Operator1/1, Relational Operator3/1
  Relational Operator3/1 -> Data Type Conversion/1
  Sum/1 -> [z_errCodeRaw]
  Relational Operator2/1 -> Debounce_Filter/1
  [z_errCodeRaw] -> Relational Operator2/1
  CTRL_COMM2/1 -> Relational Operator2/2
  Debounce_Filter/1 -> [b_errFlag]
  either_edge/1 -> Switch1/2
  Switch1/1 -> [z_errCode], UnitDelay/1
  [b_errFlag] -> b_errFlag/1
  [b_errFlag] -> either_edge/1
  [z_errCodeRaw] -> Switch1/1
  g_Hb/1 -> Sum/2
  Relational Operator1/1 -> Data Type Conversion1/1
  Data Type Conversion/1 -> Sum/1
  Data Type Conversion1/1 -> g_Hb/1
  Switch3/1 -> Data Type Conversion3/1
  Data Type Conversion3/1 -> g_Hb1/1
  g_Hb1/1 -> Sum/3
  VqFinPrev/1 -> [VqFinPrev]
  b_motStdStill/1 -> [b_motStdStill]
  [VqFinPrev] -> Abs4/1
  Abs4/1 -> Relational Operator7/1
  r_errInpTgtThres/1 -> Relational Operator7/2
  UnitDelay/1 -> [z_errCodePrev]
  [z_errCodePrev] -> Switch1/3
  [z_errCodePrev] -> Bitwise Operator1/1
  Bitwise Operator1/1 -> Switch3/2
  CTRL_COMM4/1 -> Switch3/1
  Logical Operator1/1 -> Switch3/3
  b_motEna/1 -> [b_motEna]
  Relational Operator7/1 -> Logical Operator1/3
  [b_motEna] -> Logical Operator1/1
  [b_motStdStill] -> Logical Operator1/2

== system BLDCmotor_FOC_R2017b_fixdt/BLDC_controller/F03_Control_Mode_Manager/F03_01_Mode_Transition_Calculation ==
  b_errFlag : Inport
  b_motEna : Inport  Port=2
  b_cruiseCtrlEna : Inport  Port=3
  z_ctrlModReq : Inport  Port=4
  Logical Operator1 : Logic  Operator=OR  AllPortsSameDT=off  OutDataTypeStr=boolean
  Logical Operator2 : Logic  AllPortsSameDT=off  OutDataTypeStr=boolean
  Logical Operator3 : Logic  AllPortsSameDT=off  OutDataTypeStr=boolean
  Logical Operator4 : Logic  Operator=OR  Inputs=3  AllPortsSameDT=off  OutDataTypeStr=boolean
  Logical Operator5 : Logic  Operator=NOT  AllPortsSameDT=off  OutDataTypeStr=boolean
  Logical Operator6 : Logic  Operator=OR  Inputs=3  AllPortsSameDT=off  OutDataTypeStr=boolean
  Logical Operator7 : Logic  Operator=NOT  AllPortsSameDT=off  OutDataTypeStr=boolean
  Logical Operator9 : Logic  Operator=NOT  AllPortsSameDT=off  OutDataTypeStr=boolean
  Relational Operator{1,4..5,10} (4 alike) : RelationalOperator  Operator===  OutDataTypeStr=boolean  RndMeth=Simplest  InputSameDT=off
  constant : Constant  Value=TRQ_MODE  OutDataTypeStr=Inherit: Inherit via back propagation
  constant1 : Constant  Value=SPD_MODE  OutDataTypeStr=Inherit: Inherit via back propagation
  constant5 : Constant  Value=VLT_MODE  OutDataTypeStr=Inherit: Inherit via back propagation
  constant8 : Constant  Value=OPEN_MODE  OutDataTypeStr=Inherit: Inherit via back propagation
  b_toOpen : Outport  OutputWhenDisabled=reset  InitialOutput=0  VectorParamsAs1DForOutWhenUnconnected=off
  b_toActive : Outport  Port=2  OutputWhenDisabled=reset  InitialOutput=0  VectorParamsAs1DForOutWhenUnconnected=off
  b_toSpdMod : Outport  Port=3  OutputWhenDisabled=reset  InitialOutput=0  VectorParamsAs1DForOutWhenUnconnected=off
  b_toTrqMod : Outport  Port=4  OutputWhenDisabled=reset  InitialOutput=0  VectorParamsAs1DForOutWhenUnconnected=off
  wires:
  Logical Operator3/1 -> [b_toActive]
  [z_ctrlModReq] -> Relational Operator10/1
  constant5/1 -> Relational Operator5/2
  [z_ctrlModReq] -> Relational Operator4/1
  constant/1 -> Relational Operator4/2
  constant1/1 -> Relational Operator1/2
  [z_ctrlModReq] -> Relational Operator1/1
  Relational Operator5/1 -> Logical Operator6/1
  [z_ctrlModReq] -> Relational Operator5/1
  Logical Operator9/1 -> Logical Operator3/1
  Relational Operator10/1 -> Logical Operator4/3
  [b_motEna] -> Logical Operator7/1
  [b_toOpen] -> Logical Operator9/1
  Logical Operator4/1 -> [b_toOpen]
  constant8/1 -> Relational Operator10/2
  b_motEna/1 -> [b_motEna]
  z_ctrlModReq/1 -> [z_ctrlModReq]
  [b_toOpen] -> b_toOpen/1
  [b_toActive] -> b_toActive/1
  [b_toTrqMod] -> b_toTrqMod/1
  [b_toSpdMod] -> b_toSpdMod/1
  b_errFlag/1 -> [b_errFlag]
  [b_toSpdMod] -> Logical Operator6/2
  [b_toTrqMod] -> Logical Operator6/3
  Logical Operator6/1 -> Logical Operator3/2
  Relational Operator1/1 -> Logical Operator1/1
  Logical Operator1/1 -> [b_toSpdMod]
  [b_cruiseCtrlEna] -> Logical Operator1/2
  Relational Operator4/1 -> Logical Operator2/1
  Logical Operator2/1 -> [b_toTrqMod]
  [b_cruiseCtrlEna] -> Logical Operator5/1
  Logical Operator5/1 -> Logical Operator2/2
  Logical Operator7/1 -> Logical Operator4/2
  [b_errFlag] -> Logical Operator4/1
  b_cruiseCtrlEna/1 -> [b_cruiseCtrlEna]

== system BLDCmotor_FOC_R2017b_fixdt/BLDC_controller/F03_Control_Mode_Manager/F03_03_Input_Target_Synthesis ==
  note: Input Scaling [-1000,1000] → [min,max]
  note: Final check if OPEN_MODE is requested
  z_ctrlTypSel : Inport
  z_ctrlModReq : Inport  Port=2
  z_ctrlMod : Inport  Port=3
  r_inpTgt : Inport  Port=4
  VqFinPrev : Inport  Port=5
  Data Type Conversion22 : DataTypeConversion  OutDataTypeStr=fixdt(1,16,4)  ConvertRealWorld=Stored Integer (SI)  SaturateOnIntegerOverflow=off  RndMeth=Floor
  Default_Control_Type : Subsystem
  Default_Mode : Subsystem
  FOC_Control_Type : Subsystem
  If1 : If  IfExpression=u1 == CTRL_FOC
  If2 : If  IfExpression=u1 == OPEN_MODE
  Merge : Merge
  Merge1 : Merge
  Open_Mode : Subsystem
  Saturation : Saturate  Commented=on  UpperLimit=2000  LowerLimit=-2000
  r_inpTgtSca : Outport  OutputWhenDisabled=reset  InitialOutput=0  VectorParamsAs1DForOutWhenUnconnected=off
  r_inpTgtConv : Outport  Port=2  OutputWhenDisabled=reset  InitialOutput=0  VectorParamsAs1DForOutWhenUnconnected=off
  wires:
  FOC_Control_Type/1(r_inpTgtScaFOC) -> Merge/1
  [r_inpTgtConv] -> FOC_Control_Type/1(r_inpTgtConv)
  [r_inpTgtSca] -> r_inpTgtSca/1
  If1/1 -> FOC_Control_Type/Action
  z_ctrlTypSel/1 -> [z_ctrlTypSel]
  [z_ctrlTypSel] -> If1/1
  Default_Control_Type/1(r_inpTgtScaDft) -> Merge/2
  [r_inpTgtConv] -> Default_Control_Type/1(r_inpTgtConv)
  Merge/1 -> [r_inpTgtScaRaw]
  If1/2 -> Default_Control_Type/Action
  [z_ctrlModReq] -> FOC_Control_Type/2(z_ctrlModReq)
  z_ctrlModReq/1 -> [z_ctrlModReq]
  z_ctrlMod/1 -> [z_ctrlMod]
  [z_ctrlMod] -> If2/1
  If2/1 -> Open_Mode/Action
  [VqFinPrev] -> Open_Mode/1(VqFinPrev)
  Open_Mode/1(r_inpTgtScaOpen) -> Merge1/1
  Default_Mode/1(r_inpTgtScaDft) -> Merge1/2
  Merge1/1 -> [r_inpTgtSca]
  [r_inpTgtScaRaw] -> Default_Mode/1(r_inpTgtScaRaw)
  If2/2 -> Default_Mode/Action
  VqFinPrev/1 -> [VqFinPrev]
  r_inpTgt/1 -> Data Type Conversion22/1
  Data Type Conversion22/1 -> [r_inpTgtConv]
  [r_inpTgtConv] -> r_inpTgtConv/1

== system BLDCmotor_FOC_R2017b_fixdt/BLDC_controller/F04_Field_Weakening/Field_Weakening_Enabled ==
  note: Calculate Blending Factor
  note: This blendig factor is a number between [0, 1]. It manages the Field weakening amount, ranging from 0 to a calibratable Max value.
  note: Field Weakening / Phase Advance
  z_ctrlTypSel : Inport
  r_inpTgtConv : Inport  Port=2
  n_motAbs : Inport  Port=3
  Action Port : ActionPort  ActionPortLabel=if(u1 ~= 0)
  Abs5 : Abs  OutDataTypeStr=Inherit: Inherit via back propagation  RndMeth=Zero  SaturateOnIntegerOverflow=off
  CTRL_COMM2 : Constant  Value=CTRL_FOC  OutDataTypeStr=Inherit: Inherit via back propagation
  Divide1 : Product  Inputs=*/  OutDataTypeStr=fixdt(0,16,15)  RndMeth=Simplest
  Divide14 : Product  Inputs=*/  OutDataTypeStr=fixdt(0,16,15)  RndMeth=Simplest
  Divide3 : Product  Inputs=**  RndMeth=Simplest  OutDataTypeStr=Inherit: Same as first input
  MinMax : MinMax  Function=max  Inputs=2
  MinMax1 : MinMax  Inputs=2
  Relational Operator1 : RelationalOperator  Operator===  OutDataTypeStr=boolean  RndMeth=Simplest  InputSameDT=off
  Relational Operator6 : RelationalOperator  Operator=<  OutDataTypeStr=boolean  RndMeth=Simplest  InputSameDT=off
  Saturation Dynamic : simulink/Discontinuities/Saturation Dynamic  OutMin=[]  OutMax=[]  OutDataTypeStr=Inherit: Same as second input  OutDataType=fixdt(1, 16)  OutScaling=2^-10  DoSatur=off
  Saturation Dynamic1 : simulink/Discontinuities/Saturation Dynamic  OutMin=[]  OutMax=[]  OutDataTypeStr=Inherit: Same as second input  OutDataType=fixdt(1, 16)  OutScaling=2^-10  DoSatur=off
  Sum{1..4} (4 alike) : Sum  Inputs=+-  RndMeth=Simplest  OutDataTypeStr=Inherit: Same as first input
  Switch1 : Switch  Criteria=u2 ~= 0  OutDataTypeStr=Inherit: Inherit via back propagation  RndMeth=Zero  SaturateOnIntegerOverflow=off  InputSameDT=off
  Switch2 : Switch  Criteria=u2 ~= 0  OutDataTypeStr=Inherit: Inherit via back propagation  RndMeth=Zero  SaturateOnIntegerOverflow=off  InputSameDT=off
  a_phaAdvMax : Constant  Value=a_phaAdvMax  OutDataTypeStr=fixdt(1,16,4)
  id_fieldWeakMax : Constant  Value=id_fieldWeakMax  OutDataTypeStr=fixdt(1,16,4)
  n_fieldWeakAuthHi : Constant  Value=n_fieldWeakAuthHi  OutDataTypeStr=fixdt(1,16,4)
  n_fieldWeakAuthLo : Constant  Value=n_fieldWeakAuthLo  OutDataTypeStr=fixdt(1,16,4)
  r_fieldWeakHi : Constant  Value=r_fieldWeakHi  OutDataTypeStr=fixdt(1,16,4)
  r_fieldWeakLo : Constant  Value=r_fieldWeakLo  OutDataTypeStr=fixdt(1,16,4)
  "r_fieldWeak " : Outport  VectorParamsAs1DForOutWhenUnconnected=off
  wires:
  a_phaAdvMax/1 -> Switch2/3
  [r_fieldWeak] -> "r_fieldWeak "/1
  Switch2/1 -> Divide3/1
  n_fieldWeakAuthLo/1 -> Saturation Dynamic/3, Sum4/2, Sum2/2
  CTRL_COMM2/1 -> Relational Operator1/2
  Relational Operator1/1 -> Switch2/2
  [n_motAbs] -> Saturation Dynamic/2
  n_motAbs/1 -> [n_motAbs]
  Divide14/1 -> MinMax1/2, MinMax/1, Relational Operator6/1
  Saturation Dynamic/1 -> Sum4/1
  n_fieldWeakAuthHi/1 -> Saturation Dynamic/1, Sum2/1
  Divide1/1 -> MinMax1/1, MinMax/2, Relational Operator6/2
  Sum4/1 -> Divide1/1
  [r_blendFactor] -> Divide3/2
  Sum3/1 -> Divide14/2
  id_fieldWeakMax/1 -> Switch2/1
  [r_inpTgtConv] -> Abs5/1
  Saturation Dynamic1/1 -> Sum1/1
  Sum2/1 -> Divide1/2
  Abs5/1 -> Saturation Dynamic1/2
  z_ctrlTypSel/1 -> [z_ctrlTypSel]
  r_inpTgtConv/1 -> [r_inpTgtConv]
  r_fieldWeakHi/1 -> Saturation Dynamic1/1, Sum3/1
  r_fieldWeakLo/1 -> Saturation Dynamic1/3, Sum3/2, Sum1/2
  Divide3/1 -> [r_fieldWeak]
  Sum1/1 -> Divide14/1
  [z_ctrlTypSel] -> Relational Operator1/1
  Relational Operator6/1 -> Switch1/2
  Switch1/1 -> [r_blendFactor]
  MinMax/1 -> Switch1/1
  MinMax1/1 -> Switch1/3
